simulink model "moving_platform_control"  (R2021a)
settings: Solver=ode15s  StartTime=0  StopTime=60  FixedStep=10e-3  EnableMultiTasking=on
undefined symbols (not defined in the file): C, H, initial_hight_z, L, L1, L2, L3, last_pitch, last_roll, last_u_pitch, last_u_roll, last_u_yaw, last_yaw, leg1, leg2, leg3, leg4, q0_leg1, q0_leg2, q0_leg3, q0_leg4, transl, X, Y, Z
libraries: sm_lib x44, nesl_utility x28, roblocks x8, simulink x1
settings Model: Creator=Usuário  LastModifiedBy=Usuário
settings DataIOCC: LimitDataPoints=on  MaxDataPoints=10000
settings OptimizationCC: LifeSpan=inf
settings DebuggingCC: AllowSymbolicDim=off  SFUnexpectedBacktrackingDiag=warning  SFNoUnconditionalDefaultTransitionDiag=warning  SFExecutionAtInitializationDiag=none  SFMachineParentedDataDiag=warning  ArithmeticOperatorsInVariantConditions=warning
settings SFSimCC: SimUseLocalCustomCode=off  CustomCodeUndefinedFunction=UseInterfaceOnly
settings RTWCC: RTWUseLocalCustomCode=off
settings CodeAppCC: StateflowObjectComments=on
settings GRTTargetCC: TargetLangStandard=C89/C90 (ANSI)
settings ConfigComp: CovMetricSettings=dw  CovSaveCumulativeToWorkspaceVar=on  CovSaveSingleToWorkspaceVar=on  CovExternalEMLEnable=off  CovSFcnEnable=off
settings SimscapeCC: SimscapeLogType=all  SimscapeLogSimulationStatistics=on  SimscapeLogDataHistory=10000
settings ExplorerConfigSet: InternalSimMechanicsExplorerSettings="<ExplorerConfiguration><canonicalview>planar_xy</canonicalview><AnimationSetting><BasePlaybackSpeed>1.0</BasePlaybackSpeed><PlaybackSpeedFactor>1.0</PlaybackSpeedFactor></AnimationSetting><TilePanel><TileInfo><Tiles Columns=\"1\" Count=\"1\" Rows=\"1\"><Column Weight=\"1\"/><Row Weight=\"1\"/><Tile Height=\"1\" Width=\"1\" X=\"0\" Y=\"0\"/></Tiles></TileInfo><SceneInfo><SceneViewer><BGColor><R>0.60000002384185791</R><G>0.60000002384185791</G><B>0.60000002384185791</B></BGColor><Camera><DoPerspective>off</DoPerspective><Position><X>0.649416583539183412</X><Y>-0.22604670383609643</Y><Z>4.61016604278915842</Z></Position><Center><X>0.175311972245489334</X><Y>-0.130970741281833059</Y><Z>0.0192888534073016871</Z></Center><Up><X>0.0493442595854783964</X><Y>0.998660209995804626</Y><Z>0.0155861803241310534</Z></Up><ViewLimDist>1</ViewLimDist><YLim>0.440864806646154017</YLim><XLim>0.949929693878453385</XLim></Camera></SceneViewer></SceneInfo></TilePanel><MechEditorPanel><Cameras/><GfxPanelCameraMap/><VideoCreator><PlaybackSpeedRatio>1.0</PlaybackSpeedRatio><FrameRate>30</FrameRate><VideoFormat>Motion JPEG AVI</VideoFormat><FrameSize>auto</FrameSize></VideoCreator></MechEditorPanel></ExplorerConfiguration>"

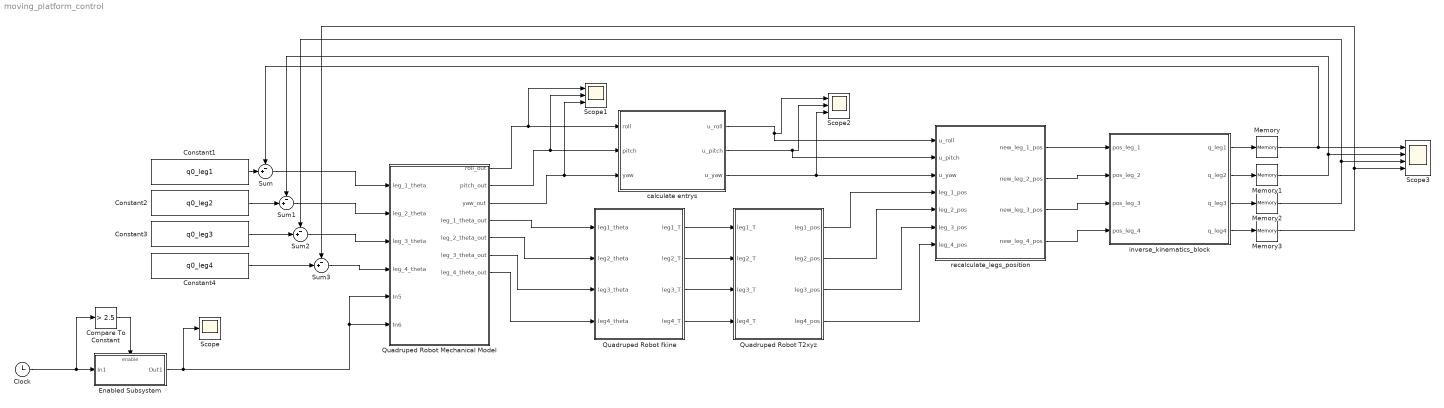
== system moving_platform_control ==
  Clock : Clock
  Compare To Constant : simulink/Logic and Bit Operations/Compare To Constant  relop=>  const=2.5  OutDataTypeStr=boolean
  Constant1 : Constant  Value=q0_leg1
  Constant2 : Constant  Value=q0_leg2
  Constant3 : Constant  Value=q0_leg3
  Constant4 : Constant  Value=q0_leg4
  Enabled Subsystem : Subsystem  TreatAsAtomicUnit=on
  Memory{,1..3} (4 alike) : Memory
  Quadruped Robot Mechanical Model : Subsystem
  Quadruped Robot T2xyz : Subsystem
  Quadruped Robot fkine : Subsystem
  Scope : Scope
  Scope1 : Scope  NumInputPorts=3
  Scope2 : Scope  NumInputPorts=3
  Scope3 : Scope  NumInputPorts=4
  Sum{,1..3} (4 alike) : Sum  Inputs=-+|
  calculate entrys : MATLAB Function  TreatAsAtomicUnit=on  mask{last_roll_param=last_roll, last_pitch_param=last_pitch, last_yaw_param=last_yaw, last_u_roll_param=last_u_roll, last_u_pitch_param=last_u_pitch, last_u_yaw_param=last_u_yaw}
      mask prompts: last_roll_param "last roll"; last_pitch_param "last pitch"; last_yaw_param "last yaw"; last_u_roll_param "last u roll"; last_u_pitch_param "last u pitch"; last_u_yaw_param "last u yaw"
  inverse_kinematics_block : MATLAB Function  TreatAsAtomicUnit=on  mask{L1=L1, L2=L2, L3=L3, p01=transl(leg1.base)', p02=transl(leg2.base)', p03=transl(leg3.base)', p04=transl(leg4.base)'}
  recalculate_legs_position : MATLAB Function  TreatAsAtomicUnit=on
  wires:
  Clock/1 -> Compare To Constant/1, Enabled Subsystem/1(In1)
  Compare To Constant/1 -> Enabled Subsystem/Enable
  Quadruped Robot Mechanical Model/2(pitch_out) -> calculate entrys/2(pitch), Scope1/2
  Quadruped Robot Mechanical Model/3(yaw_out) -> calculate entrys/3(yaw), Scope1/3
  Quadruped Robot Mechanical Model/4(leg_1_theta_out) -> Quadruped Robot fkine/1(leg1_theta)
  Quadruped Robot Mechanical Model/5(leg_2_theta_out) -> Quadruped Robot fkine/2(leg2_theta)
  Quadruped Robot Mechanical Model/6(leg_3_theta_out) -> Quadruped Robot fkine/3(leg3_theta)
  Quadruped Robot Mechanical Model/7(leg_4_theta_out) -> Quadruped Robot fkine/4(leg4_theta)
  Quadruped Robot fkine/1(leg1_T) -> Quadruped Robot T2xyz/1(leg1_T)
  Quadruped Robot fkine/2(leg2_T) -> Quadruped Robot T2xyz/2(leg2_T)
  Quadruped Robot fkine/3(leg3_T) -> Quadruped Robot T2xyz/3(leg3_T)
  Quadruped Robot fkine/4(leg4_T) -> Quadruped Robot T2xyz/4(leg4_T)
  calculate entrys/3(u_yaw) -> Scope2/3, recalculate_legs_position/3(u_yaw)
  calculate entrys/2(u_pitch) -> recalculate_legs_position/2(u_pitch), Scope2/2
  calculate entrys/1(u_roll) -> recalculate_legs_position/1(u_roll), Scope2/1
  Quadruped Robot T2xyz/1(leg1_pos) -> recalculate_legs_position/4(leg_1_pos)
  Quadruped Robot T2xyz/2(leg2_pos) -> recalculate_legs_position/5(leg_2_pos)
  Quadruped Robot T2xyz/3(leg3_pos) -> recalculate_legs_position/6(leg_3_pos)
  Quadruped Robot T2xyz/4(leg4_pos) -> recalculate_legs_position/7(leg_4_pos)
  recalculate_legs_position/1(new_leg_1_pos) -> inverse_kinematics_block/1(pos_leg_1)
  recalculate_legs_position/2(new_leg_2_pos) -> inverse_kinematics_block/2(pos_leg_2)
  recalculate_legs_position/3(new_leg_3_pos) -> inverse_kinematics_block/3(pos_leg_3)
  recalculate_legs_position/4(new_leg_4_pos) -> inverse_kinematics_block/4(pos_leg_4)
  inverse_kinematics_block/1(q_leg1) -> Memory/1
  inverse_kinematics_block/3(q_leg3) -> Memory2/1
  inverse_kinematics_block/4(q_leg4) -> Memory3/1
  inverse_kinematics_block/2(q_leg2) -> Memory1/1
  Enabled Subsystem/1(Out1) -> Scope/1, Quadruped Robot Mechanical Model/6(In6), Quadruped Robot Mechanical Model/5(In5)
  Quadruped Robot Mechanical Model/1(roll_out) -> calculate entrys/1(roll), Scope1/1
  Memory/1 -> Sum/1, Scope3/1
  Memory1/1 -> Sum1/1, Scope3/2
  Memory2/1 -> Sum2/1, Scope3/3
  Memory3/1 -> Sum3/1, Scope3/4
  Constant1/1 -> Sum/2
  Constant2/1 -> Sum1/2
  Constant3/1 -> Sum2/2
  Constant4/1 -> Sum3/2
  Sum3/1 -> Quadruped Robot Mechanical Model/4(leg_4_theta)
  Sum2/1 -> Quadruped Robot Mechanical Model/3(leg_3_theta)
  Sum1/1 -> Quadruped Robot Mechanical Model/2(leg_2_theta)
  Sum/1 -> Quadruped Robot Mechanical Model/1(leg_1_theta)

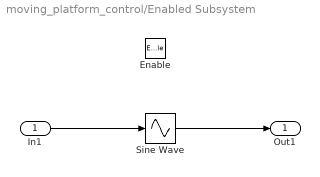
== system moving_platform_control/Enabled Subsystem ==
  In1 : Inport
  Enable : EnablePort
  Sine Wave : Sin  TimeSource=Use external signal  Amplitude=pi/18  Frequency=0.1  Phase=-0.25  SampleTime=0
  Out1 : Outport
  wires:
  In1/1 -> Sine Wave/1
  Sine Wave/1 -> Out1/1

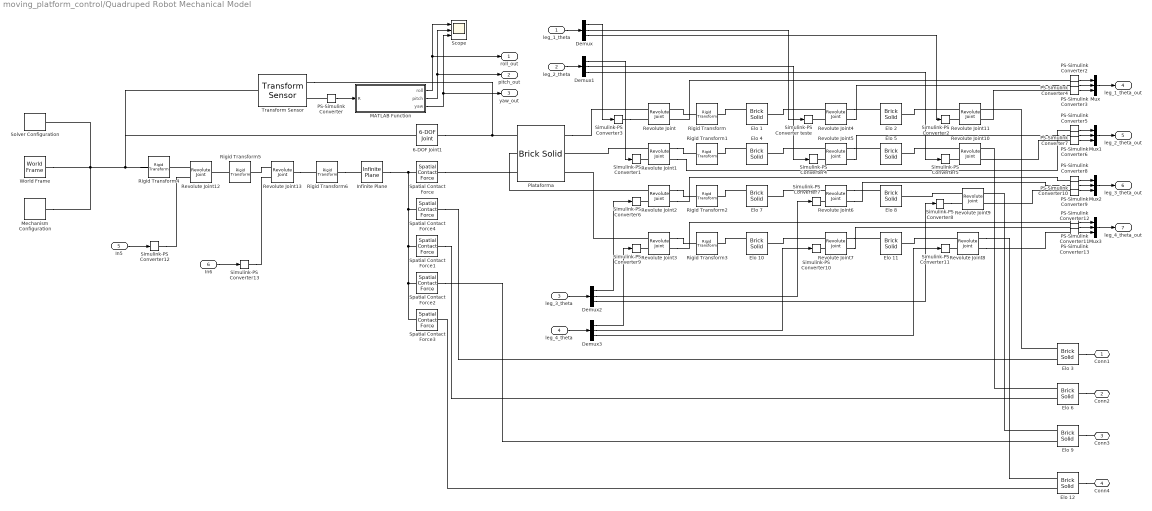
== system moving_platform_control/Quadruped Robot Mechanical Model ==
  leg_1_theta : Inport
  leg_2_theta : Inport  Port=2
  leg_3_theta : Inport  Port=3
  leg_4_theta : Inport  Port=4
  In5 : Inport  Port=5
  In6 : Inport  Port=6
  6-DOF Joint1 : sm_lib/Joints/6-DOF Joint  JointMode=Normal  SenseConstraintForce=off  SenseConstraintForceX=off  SenseConstraintForceY=off  SenseConstraintForceZ=off  SenseConstraintTorque=off  SenseConstraintTorqueX=off  SenseConstraintTorqueY=off  SenseConstraintTorqueZ=off  SenseTotalForce=off  SenseTotalForceX=off  SenseTotalForceY=off  SenseTotalForceZ=off  SenseTotalTorque=off  SenseTotalTorqueX=off  SenseTotalTorqueY=off  SenseTotalTorqueZ=off  CompositeWrenchDir=FollowerOnBase  CompositeWrenchFrame=BaseFrame  PxEquilibriumPosition=0  PxEquilibriumPositionUnits=m  PxSpringStiffness=0  PxSpringStiffnessUnits=N/m  PxDampingCoefficient=0  PxDampingCoefficientUnits=N/(m/s)  PxTorqueActuationMode=NoTorque  PxMotionActuationMode=ComputedMotion  PxSensePosition=off  PxSenseVelocity=off  PxSenseAcceleration=off  PxSenseTorqueForce=off  PxSenseLowerLimitTorqueForce=off  PxSenseUpperLimitTorqueForce=off  PxLowerLimitSpecify=off  PxLowerLimitBound=-1  PxLowerLimitBoundUnits=m  PxLowerLimitStiffness=1e6  PxLowerLimitStiffnessUnits=N/m  PxLowerLimitDamping=1e3  PxLowerLimitDampingUnits=N/(m/s)  PxLowerLimitTransitionRegionWidth=1e-4  PxLowerLimitTransitionRegionWidthUnits=m  PxUpperLimitSpecify=off  PxUpperLimitBound=1  PxUpperLimitBoundUnits=m  PxUpperLimitStiffness=1e6  PxUpperLimitStiffnessUnits=N/m  PxUpperLimitDamping=1e3  PxUpperLimitDampingUnits=N/(m/s)  PxUpperLimitTransitionRegionWidth=1e-4  PxUpperLimitTransitionRegionWidthUnits=m  PxPositionTargetSpecify=off  PxPositionTargetPriority=High  PxPositionTargetValue=0  PxPositionTargetValueUnits=m  PxVelocityTargetSpecify=off  PxVelocityTargetPriority=High  PxVelocityTargetValue=0  PxVelocityTargetValueUnits=m/s  PyEquilibriumPosition=0  PyEquilibriumPositionUnits=m  PySpringStiffness=0  PySpringStiffnessUnits=N/m  PyDampingCoefficient=0  PyDampingCoefficientUnits=N/(m/s)  PyTorqueActuationMode=NoTorque  PyMotionActuationMode=ComputedMotion  PySensePosition=off  PySenseVelocity=off  PySenseAcceleration=off  PySenseTorqueForce=off  PySenseLowerLimitTorqueForce=off  PySenseUpperLimitTorqueForce=off  PyLowerLimitSpecify=off  PyLowerLimitBound=-1  PyLowerLimitBoundUnits=m  PyLowerLimitStiffness=1e6  PyLowerLimitStiffnessUnits=N/m  PyLowerLimitDamping=1e3  PyLowerLimitDampingUnits=N/(m/s)  PyLowerLimitTransitionRegionWidth=1e-4  PyLowerLimitTransitionRegionWidthUnits=m  PyUpperLimitSpecify=off  PyUpperLimitBound=1  PyUpperLimitBoundUnits=m  PyUpperLimitStiffness=1e6  PyUpperLimitStiffnessUnits=N/m  PyUpperLimitDamping=1e3  PyUpperLimitDampingUnits=N/(m/s)  PyUpperLimitTransitionRegionWidth=1e-4  PyUpperLimitTransitionRegionWidthUnits=m  PyPositionTargetSpecify=off  PyPositionTargetPriority=High  PyPositionTargetValue=0  PyPositionTargetValueUnits=m  PyVelocityTargetSpecify=off  PyVelocityTargetPriority=High  PyVelocityTargetValue=0  PyVelocityTargetValueUnits=m/s  PzEquilibriumPosition=0  PzEquilibriumPositionUnits=m  PzSpringStiffness=0  PzSpringStiffnessUnits=N/m  PzDampingCoefficient=70  PzDampingCoefficientUnits=N/(m/s)  PzTorqueActuationMode=NoTorque  PzMotionActuationMode=ComputedMotion  PzSensePosition=off  PzSenseVelocity=off  PzSenseAcceleration=off  PzSenseTorqueForce=off  PzSenseLowerLimitTorqueForce=off  PzSenseUpperLimitTorqueForce=off  PzLowerLimitSpecify=off  PzLowerLimitBound=-1  PzLowerLimitBoundUnits=m  PzLowerLimitStiffness=1e6  PzLowerLimitStiffnessUnits=N/m  PzLowerLimitDamping=1e3  PzLowerLimitDampingUnits=N/(m/s)  PzLowerLimitTransitionRegionWidth=1e-4  PzLowerLimitTransitionRegionWidthUnits=m  PzUpperLimitSpecify=off  PzUpperLimitBound=1  PzUpperLimitBoundUnits=m  PzUpperLimitStiffness=1e6  PzUpperLimitStiffnessUnits=N/m  PzUpperLimitDamping=1e3  PzUpperLimitDampingUnits=N/(m/s)  PzUpperLimitTransitionRegionWidth=1e-4  PzUpperLimitTransitionRegionWidthUnits=m  PzPositionTargetSpecify=on  PzPositionTargetPriority=High  PzPositionTargetValue=(initial_hight_z+1)/100  PzPositionTargetValueUnits=m  PzVelocityTargetSpecify=off  PzVelocityTargetPriority=High  PzVelocityTargetValue=0  PzVelocityTargetValueUnits=m/s  SphDefPosRotationMethod=None  SphDefPosRotationAngleUnits=deg  SphDefPosRotationStandardAxis=+Z  SphDefPosRotationAngle=0.0  SphDefPosRotationArbitraryAxis=[0 0 1]  SphDefPosFollAlignAxisA=+X  SphDefPosBaseAlignAxisA=+Y  SphDefPosFollAlignAxisB=+Y  SphDefPosBaseAlignAxisB=+Z  SphDefPosRotationSequenceAxes=FollowerAxes  SphDefPosRotationSequence=XYX  SphDefPosRotationSequenceAngles=[0 0 0]  SphDefPosRotationSequenceAnglesUnits=deg  SphDefPosRotationMatrix=[1 0 0; 0 1 0; 0 0 1]  SphEqPosRotationMethod=None  SphEqPosRotationAngleUnits=deg  SphEqPosRotationStandardAxis=+Z  SphEqPosRotationAngle=0.0  SphEqPosRotationArbitraryAxis=[0 0 1]  SphEqPosFollAlignAxisA=+X  SphEqPosBaseAlignAxisA=+Y  SphEqPosFollAlignAxisB=+Y  SphEqPosBaseAlignAxisB=+Z  SphEqPosRotationSequenceAxes=FollowerAxes  SphEqPosRotationSequence=XYX  SphEqPosRotationSequenceAngles=[0 0 0]  SphEqPosRotationSequenceAnglesUnits=deg  SphEqPosRotationMatrix=[1 0 0; 0 1 0; 0 0 1]  SphSpringStiffness=0  SphSpringStiffnessUnits=N*m/deg  SphDampingCoefficient=0.7  SphDampingCoefficientUnits=N*m/(rad/s)  SphActuateTorqueX=off  SphActuateTorqueY=off  SphActuateTorqueZ=off  SphActuateTorque=off  SphTorqueActuationMode=NoTorque  SphMotionActuationMode=ComputedMotion  SphActuationFrame=BaseFrame  SphSensePosition=off  SphSenseVelocityX=off  SphSenseVelocityY=off  SphSenseVelocityZ=off  SphSenseVelocity=off  SphSenseAccelerationX=off  SphSenseAccelerationY=off  SphSenseAccelerationZ=off  SphSenseAcceleration=off  SphSenseTorqueX=off  SphSenseTorqueY=off  SphSenseTorqueZ=off  SphSenseTorqueForce=off  SphSenseLowerLimitTorqueMag=off  SphSenseUpperLimitTorqueMag=off  SphSensingFrame=BaseFrame  SphLowerLimitSpecify=off  SphLowerLimitBound=15  SphLowerLimitBoundUnits=deg  SphLowerLimitStiffness=1e4  SphLowerLimitStiffnessUnits=N*m/deg  SphLowerLimitDamping=10  SphLowerLimitDampingUnits=N*m/(deg/s)  SphLowerLimitTransitionRegionWidth=0.1  SphLowerLimitTransitionRegionWidthUnits=deg  SphUpperLimitSpecify=off  SphUpperLimitBound=45  SphUpperLimitBoundUnits=deg  SphUpperLimitStiffness=1e4  SphUpperLimitStiffnessUnits=N*m/deg  SphUpperLimitDamping=10  SphUpperLimitDampingUnits=N*m/(deg/s)  SphUpperLimitTransitionRegionWidth=0.1  SphUpperLimitTransitionRegionWidthUnits=deg  SphPositionTargetRotationMethod=None  SphPositionTargetRotationAngleUnits=deg  SphPositionTargetRotationStandardAxis=+Z  SphPositionTargetRotationAngle=0.0  SphPositionTargetRotationArbitraryAxis=[0 0 1]  SphPositionTargetFollAlignAxisA=+X  SphPositionTargetBaseAlignAxisA=+Y  SphPositionTargetFollAlignAxisB=+Y  SphPositionTargetBaseAlignAxisB=+Z  SphPositionTargetRotationSequenceAxes=FollowerAxes  SphPositionTargetRotationSequence=XYX  SphPositionTargetRotationSequenceAngles=[0 0 0]  SphPositionTargetRotationSequenceAnglesUnits=deg  SphPositionTargetRotationMatrix=[1 0 0; 0 1 0; 0 0 1]  SphPositionTargetSpecify=off  SphPositionTargetPriority=High  SphVelocityTargetValue=[0 0 0]  SphVelocityTargetValueUnits=deg/s  SphVelocityTargetSpecify=off  SphVelocityTargetPriority=High  SphVelocityTargetInFollowerFrame=on
  Demux{,1..3} (4 alike) : Demux  Outputs=3
  Elo {1,4,7,10} (4 alike) : sm_lib/Body Elements/Brick Solid  GraphicAmbientColor=[0.15 0.15 0.15 1.0]  BasedOnType=Density  BrickDimensions=[L1 H H]  BrickDimensionUnits=cm  CenterOfMass=[0 0 0]  CenterOfMassUnits=m  GraphicDiffuseColor=[1.0 0.6 0.4]  Density=1000  DensityUnits=kg/m^3  DoExposeReferenceFrame=off  GraphicEmissiveColor=[0.0 0.0 0.0 1.0]  ExportEntireGeometry=on  SerializedFrames=<Frames><Frame><Id>Frame1</Id><Value><Name>B</Name><Origin><Source>GeometricFeature</Source><FeatureName>-x surface</FeatureName></Origin><PrimaryAxis><DefinedDirection>+Y</DefinedDirection><Source>ReferenceFrame</Source><SourceDirection>+Z</SourceDirection><FeatureName></FeatureName></PrimaryAxis><SecondaryAxis><DefinedDirection>+X</DefinedDirection><Source>ReferenceFrame</Source><SourceDirection>+Y</SourceDirection><FeatureName></FeatureName></SecondaryAxis></Value></Frame><Frame><Id>Frame2</Id><Value><Name>E</Name><Origin><Source>GeometricFeature</Source><FeatureName>+x surface</FeatureName></Origin><PrimaryAxis><DefinedDirection>+Y</DefinedDirection><Source>ReferenceFrame</Source><SourceDirection>+Z</SourceDirection><FeatureName></FeatureName></PrimaryAxis><SecondaryAxis><DefinedDirection>+X</DefinedDirection><Source>ReferenceFrame</Source><SourceDirection>+Y</SourceDirection><FeatureName></FeatureName></SecondaryAxis></Value></Frame></Frames>  MarkerShape=Sphere  MarkerSize=10  GraphicType=FromGeometry  InertiaType=CalculateFromGeometry  Mass=1  MassUnits=kg  MomentsOfInertia=[1 1 1]  MomentsOfInertiaUnits=kg*m^2  GraphicOpacity=1.0  ProductsOfInertia=[0 0 0]  ProductsOfInertiaUnits=kg*m^2  GraphicShininess=75  GraphicSpecularColor=[0.5 0.5 0.5 1.0]  GraphicVisPropType=SimpleVisualProperties
  Elo {2,5,8,11} (4 alike) : sm_lib/Body Elements/Brick Solid  GraphicAmbientColor=[0.15 0.15 0.15 1.0]  BasedOnType=Density  BrickDimensions=[L2 H H]  BrickDimensionUnits=cm  CenterOfMass=[0 0 0]  CenterOfMassUnits=m  GraphicDiffuseColor=[1.0 0.4 1.0]  Density=1000  DensityUnits=kg/m^3  DoExposeReferenceFrame=off  GraphicEmissiveColor=[0.0 0.0 0.0 1.0]  ExportEntireGeometry=on  SerializedFrames=<Frames><Frame><Id>Frame1</Id><Value><Name>B</Name><Origin><Source>GeometricFeature</Source><FeatureName>-x surface</FeatureName></Origin><PrimaryAxis><DefinedDirection>+X</DefinedDirection><Source>ReferenceFrame</Source><SourceDirection>-X</SourceDirection><FeatureName></FeatureName></PrimaryAxis><SecondaryAxis><DefinedDirection>+Y</DefinedDirection><Source>ReferenceFrame</Source><SourceDirection>+Y</SourceDirection><FeatureName></FeatureName></SecondaryAxis></Value></Frame><Frame><Id>Frame2</Id><Value><Name>E</Name><Origin><Source>GeometricFeature</Source><FeatureName>+x surface</FeatureName></Origin><PrimaryAxis><DefinedDirection>+Z</DefinedDirection><Source>ReferenceFrame</Source><SourceDirection>-Z</SourceDirection><FeatureName></FeatureName></PrimaryAxis><SecondaryAxis><DefinedDirection>+X</DefinedDirection><Source>ReferenceFrame</Source><SourceDirection>-X</SourceDirection><FeatureName></FeatureName></SecondaryAxis></Value></Frame></Frames>  MarkerShape=Sphere  MarkerSize=10  GraphicType=FromGeometry  InertiaType=CalculateFromGeometry  Mass=1  MassUnits=kg  MomentsOfInertia=[1 1 1]  MomentsOfInertiaUnits=kg*m^2  GraphicOpacity=1.0  ProductsOfInertia=[0 0 0]  ProductsOfInertiaUnits=kg*m^2  GraphicShininess=75  GraphicSpecularColor=[0.5 0.5 0.5 1.0]  GraphicVisPropType=SimpleVisualProperties
  Elo {3,6,9,12} (4 alike) : sm_lib/Body Elements/Brick Solid  GraphicAmbientColor=[0.15 0.15 0.15 1.0]  BasedOnType=Density  BrickDimensions=[L3 H H]  BrickDimensionUnits=cm  CenterOfMass=[0 0 0]  CenterOfMassUnits=m  GraphicDiffuseColor=[0.4 1.0 0.2]  Density=1000  DensityUnits=kg/m^3  DoExposeReferenceFrame=off  GraphicEmissiveColor=[0.0 0.0 0.0 1.0]  ExportEntireGeometry=on  SerializedFrames=<Frames><Frame><Id>Frame1</Id><Value><Name>B</Name><Origin><Source>GeometricFeature</Source><FeatureName>-x surface</FeatureName></Origin><PrimaryAxis><DefinedDirection>+X</DefinedDirection><Source>ReferenceFrame</Source><SourceDirection>-X</SourceDirection><FeatureName></FeatureName></PrimaryAxis><SecondaryAxis><DefinedDirection>+Y</DefinedDirection><Source>ReferenceFrame</Source><SourceDirection>+Y</SourceDirection><FeatureName></FeatureName></SecondaryAxis></Value></Frame><Frame><Id>Frame2</Id><Value><Name>E</Name><Origin><Source>GeometricFeature</Source><FeatureName>+x surface</FeatureName></Origin><PrimaryAxis><DefinedDirection>+Z</DefinedDirection><Source>ReferenceFrame</Source><SourceDirection>-Z</SourceDirection><FeatureName></FeatureName></PrimaryAxis><SecondaryAxis><DefinedDirection>+X</DefinedDirection><Source>ReferenceFrame</Source><SourceDirection>-X</SourceDirection><FeatureName></FeatureName></SecondaryAxis></Value></Frame></Frames>  MarkerShape=Sphere  MarkerSize=10  GraphicType=FromGeometry  InertiaType=CalculateFromGeometry  Mass=1  MassUnits=kg  MomentsOfInertia=[1 1 1]  MomentsOfInertiaUnits=kg*m^2  GraphicOpacity=1.0  ProductsOfInertia=[0 0 0]  ProductsOfInertiaUnits=kg*m^2  GraphicShininess=75  GraphicSpecularColor=[0.5 0.5 0.5 1.0]  GraphicVisPropType=SimpleVisualProperties
  Infinite Plane : sm_lib/Curves and Surfaces/Infinite Plane  GraphicType=Rectangle  GraphicPlaneWidth=5  GraphicPlaneWidthUnits=m  GraphicPlaneHeight=5  GraphicPlaneHeightUnits=m  GraphicVisPropType=SimpleVisualProperties  GraphicDiffuseColor=[0.1843 0.3686 0.5294]  GraphicOpacity=1  GraphicSpecularColor=[0.5 0.5 0.5 1.0]  GraphicAmbientColor=[0.15 0.15 0.15 1.0]  GraphicEmissiveColor=[0.0 0.0 0.0 1.0]  GraphicShininess=75
  MATLAB Function : MATLAB Function  TreatAsAtomicUnit=on
  Mechanism Configuration : sm_lib/Utilities/Mechanism Configuration  UniformGravity=Constant  GravityVector=[0 0 -9.80665]  GravityVectorUnits=m/s^2  GravityUnits=m/s^2  LinearizationDelta=0.001  JointModeTransitionNonlinearIterations=2
  Mux{,1..3} (4 alike) : Mux  Inputs=3
  PS-Simulink Converter{,2..13} (13 alike) : nesl_utility/PS-Simulink Converter  PhysicalDomain=network_engine_domain  SubClassName=ps_output  LeftPortType=input  RightPortType=output  PseudoPeriodic=off  Frequencies=[]  Unit=inherit  AffineConversion=off
      settings: SourceProductBaseCode=PW,SS
  Plataforma : sm_lib/Body Elements/Brick Solid  GraphicAmbientColor=[0.15 0.15 0.15 1.0]  BasedOnType=Density  BrickDimensions=[C L H]  BrickDimensionUnits=cm  CenterOfMass=[0 0 0]  CenterOfMassUnits=m  GraphicDiffuseColor=[0.0 0.8 0.8]  Density=1000  DensityUnits=kg/m^3  DoExposeReferenceFrame=on  GraphicEmissiveColor=[0.0 0.0 0.0 1.0]  ExportEntireGeometry=on  SerializedFrames=<Frames><Frame><Id>Frame1</Id><Value><Name>leg_1</Name><Origin><Source>GeometricFeature</Source><FeatureName>+x +y curve</FeatureName></Origin><PrimaryAxis><DefinedDirection>+Z</DefinedDirection><Source>ReferenceFrame</Source><SourceDirection>+X</SourceDirection><FeatureName></FeatureName></PrimaryAxis><SecondaryAxis><DefinedDirection>+X</DefinedDirection><Source>ReferenceFrame</Source><SourceDirection>-Z</SourceDirection><FeatureName></FeatureName></SecondaryAxis></Value></Frame><Frame><Id>Frame2</Id><Value><Name>leg_2</Name><Origin><Source>GeometricFeature</Source><FeatureName>-x +y curve</FeatureName></Origin><PrimaryAxis><DefinedDirection>+Z</DefinedDirection><Source>ReferenceFrame</Source><SourceDirection>+X</SourceDirection><FeatureName></FeatureName></PrimaryAxis><SecondaryAxis><DefinedDirection>+X</DefinedDirection><Source>ReferenceFrame</Source><SourceDirection>-Z</SourceDirection><FeatureName></FeatureName></SecondaryAxis></Value></Frame><Frame><Id>Frame3</Id><Value><Name>leg_3</Name><Origin><Source>GeometricFeature</Source><FeatureName>+x -y curve</FeatureName></Origin><PrimaryAxis><DefinedDirection>+Z</DefinedDirection><Source>ReferenceFrame</Source><SourceDirection>+X</SourceDirection><FeatureName></FeatureName></PrimaryAxis><SecondaryAxis><DefinedDirection>+X</DefinedDirection><Source>ReferenceFrame</Source><SourceDirection>-Z</SourceDirection><FeatureName></FeatureName></SecondaryAxis></Value></Frame><Frame><Id>Frame4</Id><Value><Name>leg_4</Name><Origin><Source>GeometricFeature</Source><FeatureName>-x -y curve</FeatureName></Origin><PrimaryAxis><DefinedDirection>+Z</DefinedDirection><Source>ReferenceFrame</Source><SourceDirection>+X</SourceDirection><FeatureName></FeatureName></PrimaryAxis><SecondaryAxis><DefinedDirection>+X</DefinedDirection><Source>ReferenceFrame</Source><SourceDirection>-Z</SourceDirection><FeatureName></FeatureName></SecondaryAxis></Value></Frame></Frames>  MarkerShape=Sphere  MarkerSize=10  GraphicType=FromGeometry  InertiaType=CalculateFromGeometry  Mass=1  MassUnits=kg  MomentsOfInertia=[1 1 1]  MomentsOfInertiaUnits=kg*m^2  GraphicOpacity=1.0  ProductsOfInertia=[0 0 0]  ProductsOfInertiaUnits=kg*m^2  GraphicShininess=75  GraphicSpecularColor=[0.5 0.5 0.5 1.0]  GraphicVisPropType=SimpleVisualProperties
  Revolute Joint{,1..11} (12 alike) : sm_lib/Joints/Revolute Joint  JointMode=Normal  SenseConstraintForce=off  SenseConstraintForceX=off  SenseConstraintForceY=off  SenseConstraintForceZ=off  SenseConstraintTorque=off  SenseConstraintTorqueX=off  SenseConstraintTorqueY=off  SenseConstraintTorqueZ=off  SenseTotalForce=off  SenseTotalForceX=off  SenseTotalForceY=off  SenseTotalForceZ=off  SenseTotalTorque=off  SenseTotalTorqueX=off  SenseTotalTorqueY=off  SenseTotalTorqueZ=off  CompositeWrenchDir=FollowerOnBase  CompositeWrenchFrame=BaseFrame  EquilibriumPosition=0  EquilibriumPositionUnits=deg  SpringStiffness=contact_stiffness  SpringStiffnessUnits=N*m/deg  DampingCoefficient=contact_damping  DampingCoefficientUnits=N*m/(rad/s)  TorqueActuationMode=ComputedTorque  MotionActuationMode=InputMotion  SensePosition=on  SenseVelocity=off  SenseAcceleration=off  SenseTorqueForce=off  SenseLowerLimitTorqueForce=off  SenseUpperLimitTorqueForce=off  LowerLimitSpecify=off  LowerLimitBound=-30  LowerLimitBoundUnits=deg  LowerLimitStiffness=1e4  LowerLimitStiffnessUnits=N*m/deg  LowerLimitDamping=10  LowerLimitDampingUnits=N*m/(deg/s)  LowerLimitTransitionRegionWidth=0.1  LowerLimitTransitionRegionWidthUnits=deg  UpperLimitSpecify=off  UpperLimitBound=30  UpperLimitBoundUnits=deg  UpperLimitStiffness=1e4  UpperLimitStiffnessUnits=N*m/deg  UpperLimitDamping=10  UpperLimitDampingUnits=N*m/(deg/s)  UpperLimitTransitionRegionWidth=0.1  UpperLimitTransitionRegionWidthUnits=deg  PositionTargetSpecify=off  PositionTargetPriority=High  PositionTargetValue=0  PositionTargetValueUnits=rad  VelocityTargetSpecify=off  VelocityTargetPriority=High  VelocityTargetValue=0  VelocityTargetValueUnits=deg/s
  Revolute Joint12 : sm_lib/Joints/Revolute Joint  JointMode=Normal  SenseConstraintForce=off  SenseConstraintForceX=off  SenseConstraintForceY=off  SenseConstraintForceZ=off  SenseConstraintTorque=off  SenseConstraintTorqueX=off  SenseConstraintTorqueY=off  SenseConstraintTorqueZ=off  SenseTotalForce=off  SenseTotalForceX=off  SenseTotalForceY=off  SenseTotalForceZ=off  SenseTotalTorque=off  SenseTotalTorqueX=off  SenseTotalTorqueY=off  SenseTotalTorqueZ=off  CompositeWrenchDir=FollowerOnBase  CompositeWrenchFrame=BaseFrame  EquilibriumPosition=0  EquilibriumPositionUnits=deg  SpringStiffness=0  SpringStiffnessUnits=N*m/deg  DampingCoefficient=0  DampingCoefficientUnits=N*m/(deg/s)  TorqueActuationMode=ComputedTorque  MotionActuationMode=InputMotion  SensePosition=off  SenseVelocity=off  SenseAcceleration=off  SenseTorqueForce=off  SenseLowerLimitTorqueForce=off  SenseUpperLimitTorqueForce=off  LowerLimitSpecify=on  LowerLimitBound=-30  LowerLimitBoundUnits=deg  LowerLimitStiffness=1e4  LowerLimitStiffnessUnits=N*m/deg  LowerLimitDamping=10  LowerLimitDampingUnits=N*m/(deg/s)  LowerLimitTransitionRegionWidth=0.1  LowerLimitTransitionRegionWidthUnits=deg  UpperLimitSpecify=on  UpperLimitBound=30  UpperLimitBoundUnits=deg  UpperLimitStiffness=1e4  UpperLimitStiffnessUnits=N*m/deg  UpperLimitDamping=10  UpperLimitDampingUnits=N*m/(deg/s)  UpperLimitTransitionRegionWidth=0.1  UpperLimitTransitionRegionWidthUnits=deg  PositionTargetSpecify=off  PositionTargetPriority=High  PositionTargetValue=0  PositionTargetValueUnits=deg  VelocityTargetSpecify=off  VelocityTargetPriority=High  VelocityTargetValue=0  VelocityTargetValueUnits=deg/s
  Revolute Joint13 : sm_lib/Joints/Revolute Joint  JointMode=Normal  SenseConstraintForce=off  SenseConstraintForceX=off  SenseConstraintForceY=off  SenseConstraintForceZ=off  SenseConstraintTorque=off  SenseConstraintTorqueX=off  SenseConstraintTorqueY=off  SenseConstraintTorqueZ=off  SenseTotalForce=off  SenseTotalForceX=off  SenseTotalForceY=off  SenseTotalForceZ=off  SenseTotalTorque=off  SenseTotalTorqueX=off  SenseTotalTorqueY=off  SenseTotalTorqueZ=off  CompositeWrenchDir=FollowerOnBase  CompositeWrenchFrame=BaseFrame  EquilibriumPosition=0  EquilibriumPositionUnits=deg  SpringStiffness=0  SpringStiffnessUnits=N*m/deg  DampingCoefficient=0  DampingCoefficientUnits=N*m/(deg/s)  TorqueActuationMode=ComputedTorque  MotionActuationMode=InputMotion  SensePosition=off  SenseVelocity=off  SenseAcceleration=off  SenseTorqueForce=off  SenseLowerLimitTorqueForce=off  SenseUpperLimitTorqueForce=off  LowerLimitSpecify=on  LowerLimitBound=-30  LowerLimitBoundUnits=deg  LowerLimitStiffness=1e4  LowerLimitStiffnessUnits=N*m/deg  LowerLimitDamping=10  LowerLimitDampingUnits=N*m/(deg/s)  LowerLimitTransitionRegionWidth=0.1  LowerLimitTransitionRegionWidthUnits=deg  UpperLimitSpecify=on  UpperLimitBound=30  UpperLimitBoundUnits=deg  UpperLimitStiffness=1e4  UpperLimitStiffnessUnits=N*m/deg  UpperLimitDamping=10  UpperLimitDampingUnits=N*m/(deg/s)  UpperLimitTransitionRegionWidth=0.1  UpperLimitTransitionRegionWidthUnits=deg  PositionTargetSpecify=off  PositionTargetPriority=High  PositionTargetValue=0  PositionTargetValueUnits=deg  VelocityTargetSpecify=off  VelocityTargetPriority=High  VelocityTargetValue=0  VelocityTargetValueUnits=deg/s
  Rigid Transform : sm_lib/Frames and Transforms/Rigid Transform  TranslationMethod=None  TranslationStandardOffset=0  TranslationLengthUnit=m  TranslationStandardAxis=+Z  TranslationCartesianOffset=[0 0 0]  TranslationROffset=0  TranslationROffsetUnits=m  TranslationZOffset=0  TranslationZOffsetUnits=m  TranslationThetaOffset=0  TranslationThetaOffsetUnits=deg  RotationMethod=RotationMatrix  RotationAngleUnits=deg  RotationStandardAxis=+Z  RotationAngle=0.0  RotationArbitraryAxis=[0 0 1]  FollAlignAxisA=+X  BaseAlignAxisA=+Y  FollAlignAxisB=+Y  BaseAlignAxisB=+Z  RotationSequenceAxes=FollowerAxes  RotationSequence=XYX  RotationSequenceAngles=[0 0 0]  RotationSequenceAnglesUnits=deg  RotationMatrix=[-1 0 0; 0 0 1; 0 1 0]
  Rigid Transform1 : sm_lib/Frames and Transforms/Rigid Transform  TranslationMethod=None  TranslationStandardOffset=0  TranslationLengthUnit=m  TranslationStandardAxis=+Z  TranslationCartesianOffset=[0 0 0]  TranslationROffset=0  TranslationROffsetUnits=m  TranslationZOffset=0  TranslationZOffsetUnits=m  TranslationThetaOffset=0  TranslationThetaOffsetUnits=deg  RotationMethod=RotationMatrix  RotationAngleUnits=deg  RotationStandardAxis=+Z  RotationAngle=0.0  RotationArbitraryAxis=[0 0 1]  FollAlignAxisA=+X  BaseAlignAxisA=+Y  FollAlignAxisB=+Y  BaseAlignAxisB=+Z  RotationSequenceAxes=FollowerAxes  RotationSequence=XYX  RotationSequenceAngles=[0 0 0]  RotationSequenceAnglesUnits=deg  RotationMatrix=[-1 0 0; 0 0 1; 0 1 0]
  Rigid Transform2 : sm_lib/Frames and Transforms/Rigid Transform  TranslationMethod=None  TranslationStandardOffset=0  TranslationLengthUnit=m  TranslationStandardAxis=+Z  TranslationCartesianOffset=[0 0 0]  TranslationROffset=0  TranslationROffsetUnits=m  TranslationZOffset=0  TranslationZOffsetUnits=m  TranslationThetaOffset=0  TranslationThetaOffsetUnits=deg  RotationMethod=RotationMatrix  RotationAngleUnits=deg  RotationStandardAxis=+Z  RotationAngle=0.0  RotationArbitraryAxis=[0 0 1]  FollAlignAxisA=+X  BaseAlignAxisA=+Y  FollAlignAxisB=+Y  BaseAlignAxisB=+Z  RotationSequenceAxes=FollowerAxes  RotationSequence=XYX  RotationSequenceAngles=[0 0 0]  RotationSequenceAnglesUnits=deg  RotationMatrix=[-1 0 0; 0 0 -1; 0 -1 0]
  Rigid Transform3 : sm_lib/Frames and Transforms/Rigid Transform  TranslationMethod=None  TranslationStandardOffset=0  TranslationLengthUnit=m  TranslationStandardAxis=+Z  TranslationCartesianOffset=[0 0 0]  TranslationROffset=0  TranslationROffsetUnits=m  TranslationZOffset=0  TranslationZOffsetUnits=m  TranslationThetaOffset=0  TranslationThetaOffsetUnits=deg  RotationMethod=RotationMatrix  RotationAngleUnits=deg  RotationStandardAxis=+Z  RotationAngle=0.0  RotationArbitraryAxis=[0 0 1]  FollAlignAxisA=+X  BaseAlignAxisA=+Y  FollAlignAxisB=+Y  BaseAlignAxisB=+Z  RotationSequenceAxes=FollowerAxes  RotationSequence=XYX  RotationSequenceAngles=[0 0 0]  RotationSequenceAnglesUnits=deg  RotationMatrix=[-1 0 0; 0 0 -1; 0 -1 0]
  Rigid Transform4 : sm_lib/Frames and Transforms/Rigid Transform  TranslationMethod=None  TranslationStandardOffset=0  TranslationLengthUnit=m  TranslationStandardAxis=+Z  TranslationCartesianOffset=[0 0 0]  TranslationROffset=0  TranslationROffsetUnits=m  TranslationZOffset=0  TranslationZOffsetUnits=m  TranslationThetaOffset=0  TranslationThetaOffsetUnits=deg  RotationMethod=RotationMatrix  RotationAngleUnits=deg  RotationStandardAxis=+Z  RotationAngle=0.0  RotationArbitraryAxis=[0 0 1]  FollAlignAxisA=+X  BaseAlignAxisA=+Y  FollAlignAxisB=+Y  BaseAlignAxisB=+Z  RotationSequenceAxes=FollowerAxes  RotationSequence=XYX  RotationSequenceAngles=[0 0 0]  RotationSequenceAnglesUnits=deg  RotationMatrix=[0 0 1; 1 0 0; 0 1 0]
  Rigid Transform5 : sm_lib/Frames and Transforms/Rigid Transform  TranslationMethod=None  TranslationStandardOffset=0  TranslationLengthUnit=m  TranslationStandardAxis=+Z  TranslationCartesianOffset=[0 0 0]  TranslationROffset=0  TranslationROffsetUnits=m  TranslationZOffset=0  TranslationZOffsetUnits=m  TranslationThetaOffset=0  TranslationThetaOffsetUnits=deg  RotationMethod=RotationMatrix  RotationAngleUnits=deg  RotationStandardAxis=+Z  RotationAngle=0.0  RotationArbitraryAxis=[0 0 1]  FollAlignAxisA=+X  BaseAlignAxisA=+Y  FollAlignAxisB=+Y  BaseAlignAxisB=+Z  RotationSequenceAxes=FollowerAxes  RotationSequence=XYX  RotationSequenceAngles=[0 0 0]  RotationSequenceAnglesUnits=deg  RotationMatrix=[0 0 1; 1 0 0; 0 1 0]
  Rigid Transform6 : sm_lib/Frames and Transforms/Rigid Transform  TranslationMethod=None  TranslationStandardOffset=0  TranslationLengthUnit=m  TranslationStandardAxis=+Z  TranslationCartesianOffset=[0 0 0]  TranslationROffset=0  TranslationROffsetUnits=m  TranslationZOffset=0  TranslationZOffsetUnits=m  TranslationThetaOffset=0  TranslationThetaOffsetUnits=deg  RotationMethod=RotationMatrix  RotationAngleUnits=deg  RotationStandardAxis=+Z  RotationAngle=0.0  RotationArbitraryAxis=[0 0 1]  FollAlignAxisA=+X  BaseAlignAxisA=+Y  FollAlignAxisB=+Y  BaseAlignAxisB=+Z  RotationSequenceAxes=FollowerAxes  RotationSequence=XYX  RotationSequenceAngles=[0 0 0]  RotationSequenceAnglesUnits=deg  RotationMatrix=[0 0 1; 1 0 0; 0 1 0]
  Scope : Scope  NumInputPorts=3
  Simulink-PS Converter teste : nesl_utility/Simulink-PS Converter  PhysicalDomain=network_engine_domain  SubClassName=ps_input  LeftPortType=input  RightPortType=output  PseudoPeriodic=off  Frequencies=[]  NoiseDistribution=none  NoiseParameters=[]  Unit=1  AffineConversion=off  FilteringAndDerivatives=filter  SimscapeFilterOrder=2  InputFilterTimeConstant=0.001  UdotUserProvided=0
      settings: SourceProductBaseCode=PW,SS
  Simulink-PS Converter{1..13} (13 alike) : nesl_utility/Simulink-PS Converter  PhysicalDomain=network_engine_domain  SubClassName=ps_input  LeftPortType=input  RightPortType=output  PseudoPeriodic=off  Frequencies=[]  NoiseDistribution=none  NoiseParameters=[]  Unit=1  AffineConversion=off  FilteringAndDerivatives=filter  SimscapeFilterOrder=2  InputFilterTimeConstant=0.001  UdotUserProvided=0
      settings: SourceProductBaseCode=PW,SS
  Solver Configuration : nesl_utility/Solver Configuration  PhysicalDomain=network_engine_domain  SubClassName=solver  LeftPortType=input  RightPortType=generic  Tones=[]  Harmonics=[]  SimulateNoise=off  Profile=off  UseLocalSampling=off  EnableSwitchedLinearOptims=on  FrequencyDomain=off  UseCCode=off  RelTol=0.001  AbsTol=1e-06  MinStep=1e-09  ToWorkspace=off  RevertToSquareIcSolve=off  NumHomotopyIterations=100  PhasorMode=off  PhasorModeNumHarmonics=1  DoDC=off  ResidualTolerance=1e-09  UseLocalSolver=off  LocalSolverChoice=NE_BACKWARD_EULER_ADVANCER  LocalSolverSampleTime=0.001  DoFixedCost=off  MaxNonlinIter=3  MaxModeIter=2  ComputeImpulses=off  ImpulseIterations=2  LinearAlgebra=Sparse  EquationFormulation=NE_TIME_EF  DelaysMemoryBudget=1024  AutomaticFiltering=on  FilteringTimeConstant=0.001  PartitionStorageMethod=AS_NEEDED  PartitionMemoryBudget=1024  PartitionMethod=FAST
      settings: SourceProductBaseCode=PW,SS
  Spatial Contact Force{,1..4} (5 alike) : sm_lib/Forces and Torques/Spatial Contact Force  CoefficientOfDynamicFriction=dynamic_friction  CoefficientOfStaticFriction=static_friction  SenseContactBaseRotation=off  SenseContactBaseTranslation=off  NormalDamping=contact_damping  NormalDampingUnits=N/(m/s)  SenseContactFollowerRotation=off  SenseContactFollowerTranslation=off  SenseContactSignal=off  NormalStiffness=contact_stiffness  NormalStiffnessUnits=N/m  FrictionalCriticalVelocity=critical_velocity  FrictionalCriticalVelocityUnits=m/s  ZeroCrossDetectContactStartAndEnd=off  FrictionType=SmoothStickSlip  SenseFrictionalForceMagnitude=off  SenseNormalForceMagnitude=off  NormalForceType=SmoothSpringDamper  SenseNormalVelocity=off  SenseSeparationDistance=off  SenseTangentialVelocity=off  SenseTangentialVelocityMagnitude=off  NormalTransitionRegionWidth=1e-4  NormalTransitionRegionWidthUnits=m
  Transform Sensor : sm_lib/Frames and Transforms/Transform Sensor  MeasurementFrame=World  SenseAngle=off  SenseAxis=off  SenseAngle1=off  SenseAngle2=off  SenseAngle3=off  SenseQ=off  SenseR=on  SenseOmegaX=off  SenseOmegaY=off  SenseOmegaZ=off  SenseOmega1=off  SenseOmega2=off  SenseOmega3=off  SenseQDot=off  SenseRDot=off  SenseAlphaX=off  SenseAlphaY=off  SenseAlphaZ=off  SenseAlpha1=off  SenseAlpha2=off  SenseAlpha3=off  SenseQDDot=off  SenseRDDot=off  SenseX=off  SenseY=off  SenseZ=off  SenseRad=off  SenseAzim=off  SenseDist=off  SenseInc=off  SenseXDot=off  SenseYDot=off  SenseZDot=off  SenseRadDot=off  SenseAzimDot=off  SenseDistDot=off  SenseIncDot=off  SenseXDDot=off  SenseYDDot=off  SenseZDDot=off  SenseRadDDot=off  SenseAzimDDot=off  SenseDistDDot=off  SenseIncDDot=off
  World Frame : sm_lib/Frames and Transforms/World Frame
  Conn1 : PMIOPort  Side=Right
  Conn2 : PMIOPort  Port=2  Side=Right
  Conn3 : PMIOPort  Port=3  Side=Right
  Conn4 : PMIOPort  Port=4  Side=Right
  roll_out : Outport
  pitch_out : Outport  Port=2
  yaw_out : Outport  Port=3
  leg_1_theta_out : Outport  Port=4
  leg_2_theta_out : Outport  Port=5
  leg_3_theta_out : Outport  Port=6
  leg_4_theta_out : Outport  Port=7
  wires:
  Demux2/2 -> Simulink-PS Converter7/1
  Demux1/1 -> Simulink-PS Converter1/1
  Demux2/3 -> Simulink-PS Converter8/1
  Demux3/2 -> Simulink-PS Converter10/1
  Demux/3 -> Simulink-PS Converter2/1
  Demux3/3 -> Simulink-PS Converter11/1
  Demux1/2 -> Simulink-PS Converter4/1
  Demux1/3 -> Simulink-PS Converter5/1
  Demux2/1 -> Simulink-PS Converter6/1
  Demux/2 -> Simulink-PS Converter teste/1
  Demux3/1 -> Simulink-PS Converter9/1
  leg_1_theta/1 -> Demux/1
  Demux/1 -> Simulink-PS Converter3/1
  leg_2_theta/1 -> Demux1/1
  leg_3_theta/1 -> Demux2/1
  leg_4_theta/1 -> Demux3/1
  In5/1 -> Simulink-PS Converter12/1
  In6/1 -> Simulink-PS Converter13/1
  MATLAB Function/1(roll) -> Scope/1, roll_out/1
  MATLAB Function/2(pitch) -> Scope/2, pitch_out/1
  MATLAB Function/3(yaw) -> Scope/3, yaw_out/1
  PS-Simulink Converter/1 -> MATLAB Function/1(R)
  PS-Simulink Converter2/1 -> Mux/1
  PS-Simulink Converter3/1 -> Mux/2
  PS-Simulink Converter4/1 -> Mux/3
  Mux/1 -> leg_1_theta_out/1
  PS-Simulink Converter7/1 -> Mux1/3
  PS-Simulink Converter6/1 -> Mux1/2
  Mux1/1 -> leg_2_theta_out/1
  PS-Simulink Converter5/1 -> Mux1/1
  PS-Simulink Converter10/1 -> Mux2/3
  PS-Simulink Converter9/1 -> Mux2/2
  Mux2/1 -> leg_3_theta_out/1
  PS-Simulink Converter8/1 -> Mux2/1
  PS-Simulink Converter13/1 -> Mux3/3
  PS-Simulink Converter12/1 -> Mux3/2
  Mux3/1 -> leg_4_theta_out/1
  PS-Simulink Converter11/1 -> Mux3/1
  connections:
  Revolute Joint3/LConn2 -- Simulink-PS Converter9/RConn1
  Elo 9/LConn1 -- Revolute Joint9/RConn1
  Revolute Joint7/LConn1 -- Elo 10/RConn1
  Elo 12/RConn1 -- Conn4/RConn1
  Elo 9/RConn1 -- Conn3/RConn1
  Revolute Joint3/LConn1 -- Plataforma/LConn3
  Revolute Joint11/LConn1 -- Elo 2/RConn1
  Revolute Joint2/LConn1 -- Plataforma/RConn2
  Revolute Joint6/RConn1 -- Elo 8/LConn1
  Revolute Joint10/LConn2 -- Simulink-PS Converter5/RConn1
  Revolute Joint7/RConn1 -- Elo 11/LConn1
  Revolute Joint8/LConn2 -- Simulink-PS Converter11/RConn1
  Elo 6/RConn1 -- Conn2/RConn1
  Elo 1/LConn1 -- Rigid Transform/RConn1
  Revolute Joint6/LConn1 -- Elo 7/RConn1
  Elo 6/LConn1 -- Revolute Joint10/RConn1
  Revolute Joint8/LConn1 -- Elo 11/RConn1
  Rigid Transform/LConn1 -- Revolute Joint/RConn1
  Revolute Joint2/RConn1 -- Rigid Transform2/LConn1
  Revolute Joint1/LConn1 -- Plataforma/LConn2
  Revolute Joint10/LConn1 -- Elo 5/RConn1
  Elo 7/LConn1 -- Rigid Transform2/RConn1
  Revolute Joint5/LConn1 -- Elo 4/RConn1
  Revolute Joint8/RConn1 -- Elo 12/LConn1
  Plataforma/LConn1 -- Revolute Joint/LConn1
  Elo 4/LConn1 -- Rigid Transform1/RConn1
  Elo 3/RConn1 -- Conn1/RConn1
  Elo 3/LConn1 -- Revolute Joint11/RConn1
  Revolute Joint7/LConn2 -- Simulink-PS Converter10/RConn1
  Revolute Joint4/RConn1 -- Elo 2/LConn1
  Revolute Joint11/LConn2 -- Simulink-PS Converter2/RConn1
  Revolute Joint4/LConn1 -- Elo 1/RConn1
  Revolute Joint1/RConn1 -- Rigid Transform1/LConn1
  Revolute Joint3/RConn1 -- Rigid Transform3/LConn1
  Elo 10/LConn1 -- Rigid Transform3/RConn1
  Revolute Joint5/LConn2 -- Simulink-PS Converter4/RConn1
  Revolute Joint5/RConn1 -- Elo 5/LConn1
  Revolute Joint2/LConn2 -- Simulink-PS Converter6/RConn1
  Revolute Joint1/LConn2 -- Simulink-PS Converter1/RConn1
  Revolute Joint6/LConn2 -- Simulink-PS Converter7/RConn1
  Simulink-PS Converter8/RConn1 -- Revolute Joint9/LConn2
  World Frame/RConn1 -- Mechanism Configuration/RConn1 -- 6-DOF Joint1/LConn1 -- Transform Sensor/LConn1 -- Rigid Transform4/LConn1 -- Solver Configuration/RConn1
  Infinite Plane/RConn1 -- Spatial Contact Force4/LConn1 -- Spatial Contact Force1/LConn1 -- Spatial Contact Force2/LConn1 -- Spatial Contact Force3/LConn1 -- Spatial Contact Force/LConn1
  Spatial Contact Force/RConn1 -- Plataforma/RConn3
  Plataforma/RConn1 -- Transform Sensor/RConn1 -- 6-DOF Joint1/RConn1
  Spatial Contact Force4/RConn1 -- Elo 3/LConn2
  Spatial Contact Force1/RConn1 -- Elo 6/LConn2
  Spatial Contact Force2/RConn1 -- Elo 9/LConn2
  Elo 12/LConn2 -- Spatial Contact Force3/RConn1
  Simulink-PS Converter12/RConn1 -- Revolute Joint12/LConn2
  Revolute Joint12/LConn1 -- Rigid Transform4/RConn1
  Rigid Transform5/LConn1 -- Revolute Joint12/RConn1
  Revolute Joint13/LConn1 -- Rigid Transform5/RConn1
  Rigid Transform6/RConn1 -- Infinite Plane/LConn1
  Revolute Joint13/RConn1 -- Rigid Transform6/LConn1
  Simulink-PS Converter13/RConn1 -- Revolute Joint13/LConn2
  PS-Simulink Converter/LConn1 -- Transform Sensor/RConn2
  PS-Simulink Converter2/LConn1 -- Revolute Joint/RConn2
  Revolute Joint4/RConn2 -- PS-Simulink Converter3/LConn1
  PS-Simulink Converter4/LConn1 -- Revolute Joint11/RConn2
  Revolute Joint1/RConn2 -- PS-Simulink Converter5/LConn1
  Revolute Joint5/RConn2 -- PS-Simulink Converter6/LConn1
  PS-Simulink Converter7/LConn1 -- Revolute Joint10/RConn2
  Revolute Joint2/RConn2 -- PS-Simulink Converter8/LConn1
  Revolute Joint6/RConn2 -- PS-Simulink Converter9/LConn1
  PS-Simulink Converter10/LConn1 -- Revolute Joint9/RConn2
  Revolute Joint3/RConn2 -- PS-Simulink Converter11/LConn1
  Revolute Joint7/RConn2 -- PS-Simulink Converter12/LConn1
  Revolute Joint8/RConn2 -- PS-Simulink Converter13/LConn1
  Simulink-PS Converter3/RConn1 -- Revolute Joint/LConn2
  Revolute Joint4/LConn2 -- Simulink-PS Converter teste/RConn1
  Revolute Joint9/LConn1 -- Elo 8/RConn1

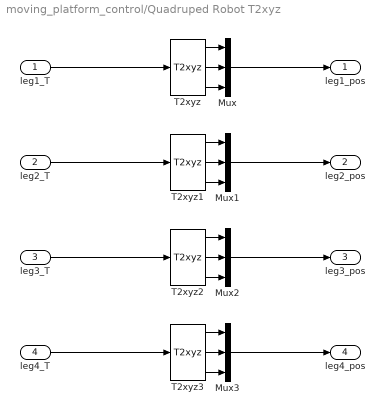
== system moving_platform_control/Quadruped Robot T2xyz ==
  leg1_T : Inport
  leg2_T : Inport  Port=2
  leg3_T : Inport  Port=3
  leg4_T : Inport  Port=4
  Mux{,1..3} (4 alike) : Mux  Inputs=3
  T2xyz{,1..3} (4 alike) : roblocks/Toolbox/T2xyz
  leg1_pos : Outport
  leg2_pos : Outport  Port=2
  leg3_pos : Outport  Port=3
  leg4_pos : Outport  Port=4
  wires:
  leg2_T/1 -> T2xyz1/1
  Mux/1 -> leg1_pos/1
  leg1_T/1 -> T2xyz/1
  Mux1/1 -> leg2_pos/1
  Mux2/1 -> leg3_pos/1
  leg4_T/1 -> T2xyz3/1
  leg3_T/1 -> T2xyz2/1
  Mux3/1 -> leg4_pos/1
  T2xyz/1 -> Mux/1
  T2xyz/2 -> Mux/2
  T2xyz/3 -> Mux/3
  T2xyz1/1 -> Mux1/1
  T2xyz1/2 -> Mux1/2
  T2xyz1/3 -> Mux1/3
  T2xyz2/1 -> Mux2/1
  T2xyz2/2 -> Mux2/2
  T2xyz2/3 -> Mux2/3
  T2xyz3/3 -> Mux3/3
  T2xyz3/1 -> Mux3/1
  T2xyz3/2 -> Mux3/2

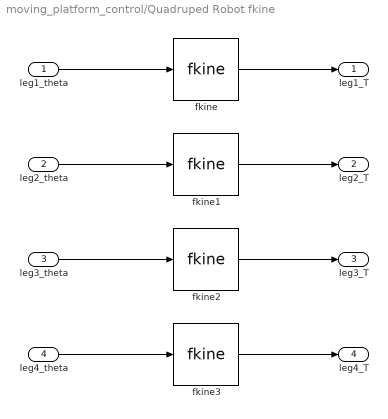
== system moving_platform_control/Quadruped Robot fkine ==
  leg1_theta : Inport
  leg2_theta : Inport  Port=2
  leg3_theta : Inport  Port=3
  leg4_theta : Inport  Port=4
  fkine : roblocks/Arm/fkine  robot=leg1
  fkine1 : roblocks/Arm/fkine  robot=leg2
  fkine2 : roblocks/Arm/fkine  robot=leg3
  fkine3 : roblocks/Arm/fkine  robot=leg4
  leg1_T : Outport
  leg2_T : Outport  Port=2
  leg3_T : Outport  Port=3
  leg4_T : Outport  Port=4
  wires:
  leg2_theta/1 -> fkine1/1
  fkine/1 -> leg1_T/1
  leg1_theta/1 -> fkine/1
  fkine1/1 -> leg2_T/1
  fkine2/1 -> leg3_T/1
  leg4_theta/1 -> fkine3/1
  leg3_theta/1 -> fkine2/1
  fkine3/1 -> leg4_T/1

== matlab function moving_platform_control/calculate entrys ==
  data: roll input; u_roll output; pitch input; yaw input; u_pitch output; u_yaw output; last_roll_param parameter; last_pitch_param parameter; last_yaw_param parameter; last_u_roll_param parameter; last_u_pitch_param parameter; last_u_yaw_param parameter
function [u_roll, u_pitch, u_yaw] = calculate_entrys(roll, pitch, yaw, ...
    last_roll_param, last_pitch_param, last_yaw_param, ...
last_u_roll_param, last_u_pitch_param, last_u_yaw_param)

Kp = 10;   % Ganho proporcional
Kd = 5;   % Ganho derivativo
I_roll = 0;
I_pitch = 0;
I_yaw = 0;

% Cálculo dos sinais de controle (equação original)
u_roll = (1 - Kp)*last_u_roll_param + Kp*roll + I_roll + Kd*(roll - last_roll_param);
u_pitch = (1 - Kp)*last_u_pitch_param + Kp*pitch + I_pitch + Kd*(pitch - last_pitch_param);
u_yaw = (1 - Kp)*last_u_yaw_param + Kp*yaw + I_yaw + Kd*(yaw - last_yaw_param);

% teste ######################
u_roll = 0;
u_pitch = 0;
u_yaw = 0;
% teste ######################

% Verificação individual: se o valor for pequeno, zera
% if abs(u_roll) < 1e-3
%     u_roll = 0;
% end
% if abs(u_pitch) < 1e-3
%     u_pitch = 0;
% end
% if abs(u_yaw) < 1e-3
%     u_yaw = 0;
% end

% Atualização dos valores persistentes para próxima iteração
last_roll_param = roll;
last_pitch_param = pitch;
last_yaw_param = yaw;
last_u_roll_param = u_roll;
last_u_pitch_param = u_pitch;
last_u_yaw_param = u_yaw;
end

== matlab function moving_platform_control/Quadruped Robot Mechanical Model/MATLAB Function ==
  data: R input; roll output; pitch output; yaw output
function [roll, pitch, yaw] = rotm2eul_custom(R)
% R é uma matriz 3x3 de rotação
% euler = [yaw, pitch, roll]

euler = rotm2eul(R, 'ZYX');
roll = euler(3);
pitch = euler(2);
yaw = euler(1);
end

== matlab function moving_platform_control/recalculate_legs_position ==
  data: u_roll input; new_leg_1_pos output; u_pitch input; u_yaw input; leg_1_pos input; leg_2_pos input; leg_3_pos input; leg_4_pos input; new_leg_2_pos output; new_leg_3_pos output; new_leg_4_pos output
function [new_leg_1_pos, new_leg_2_pos, new_leg_3_pos, new_leg_4_pos] = recalculate_legs_position(u_roll, u_pitch, u_yaw, leg_1_pos, leg_2_pos, leg_3_pos, leg_4_pos)

C = 80; % Comprimento
L = 30; % Largura

Rworld_base = rotx(rad2deg(u_roll))*roty(rad2deg(u_pitch))*rotz(rad2deg(u_yaw));

pb01 = [0, 0, 1, +C/2; 0, 1, 0, +L/2; -1, 0, 0, 0; 0, 0, 0, 1]; % centro -> perna dianteira/esquerda
pb02 = [0, 0, 1, -C/2; 0, 1, 0, +L/2; -1, 0, 0, 0; 0, 0, 0, 1]; % centro -> perna traseira/esquerda
pb03 = [0, 0, 1, +C/2; 0, 1, 0, -L/2; -1, 0, 0, 0; 0, 0, 0, 1]; % centro -> perna dianteira/direita
pb04 = [0, 0, 1, -C/2; 0, 1, 0, -L/2; -1, 0, 0, 0; 0, 0, 0, 1]; % centro -> perna traseira/direita

pos_base_1 = pb01(1:3,4);
pos_base_2 = pb02(1:3,4);
pos_base_3 = pb03(1:3,4);
pos_base_4 = pb04(1:3,4);

new_leg_1_pos = Rworld_base \ (leg_1_pos - pos_base_1) + pos_base_1;
new_leg_2_pos = Rworld_base \ (leg_2_pos - pos_base_2) + pos_base_2;
new_leg_3_pos = Rworld_base \ (leg_3_pos - pos_base_3) + pos_base_3;
new_leg_4_pos = Rworld_base \ (leg_4_pos - pos_base_4) + pos_base_4;

== matlab function moving_platform_control/inverse_kinematics_block ==
  data: pos_leg_1 input; q_leg1 output; pos_leg_2 input; pos_leg_3 input; pos_leg_4 input; q_leg2 output; q_leg3 output; q_leg4 output; L1 parameter; L2 parameter; L3 parameter; p01 parameter; p02 parameter; p03 parameter; p04 parameter
function [q_leg1, q_leg2, q_leg3, q_leg4] = inverse_kinematics_block(pos_leg_1, pos_leg_2, pos_leg_3, pos_leg_4, L1, L2, L3, p01, p02, p03, p04)

    % Agrupamento das pernas e posições
    p0s = {p01, p02, p03, p04};
    positions = {pos_leg_1, pos_leg_2, pos_leg_3, pos_leg_4};
    
    q_all = cell(1,4); % para armazenar os vetores de juntas das 4 pernas

    for i = 1:4
        pos = positions{i};
        p0 = p0s{i}; % Origem da base da perna no frame do corpo (CM)
        
        % Cálculo no plano Y-Z (visão frontal)
        n = abs(pos(2) - p0(2)); % y - y0
        m = abs(pos(3) - p0(3)); % z - z0
        p = sqrt(n*n + m*m);     % hipotenusa
        
        beta = atan(n/m);
        tau = asin(L1 / p);
        theta_1 = beta - tau;
        
        % Cálculo no plano X-Z (visão lateral)
        R = sqrt(p*p - L1*L1);
        b = pos(1) - p0(1);
        c = R;
        a = sqrt(b*b + c*c);
        phi = asin(b / a);
        
        alpha = acos((a*a + L2*L2 - L3*L3) / (2 * a * L2));

        theta_2 = alpha - phi;
        theta_3 = -pi + acos((L2*L2 + L3*L3 - a*a) / (2 * L2 * L3));
        
        q = [theta_1; theta_2; theta_3];
        
        % Invertemos o sinal das juntas para as pernas 3 e 4
        if i == 3 || i == 4
            q = -q;
        end
        
        % Zera componentes muito pequenas individualmente
%         if abs(q(1)) < 1e-3
%             q(1) = 0;
%         end
%         if abs(q(2)) < 1e-3
%             q(2) = 0;
%         end
%         if abs(q(3)) < 1e-3
%             q(3) = 0;
%         end
        
        q_all{i} = q;
    end
    
    % Atribuição às variáveis de saída
    q_leg1 = q_all{1};
    q_leg2 = q_all{2};
    q_leg3 = q_all{3};
    q_leg4 = q_all{4};
end
